simulink model "algeEquation"  (R2024b)
settings: Solver=VariableStepAuto  StartTime=0.0  StopTime=10.0  RelTol=1e-3
values from neighbouring files (symbols this model uses):
  m = input("enter the value for slop(m): ")    [algeEquMfile.m]
libraries: simulink x1
settings Model: Creator=admin  LastModifiedBy=admin

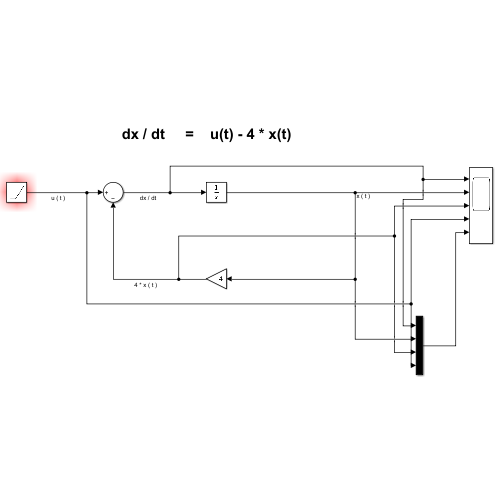
[thumbnail: Simulink's stored preview of the top-level diagram]
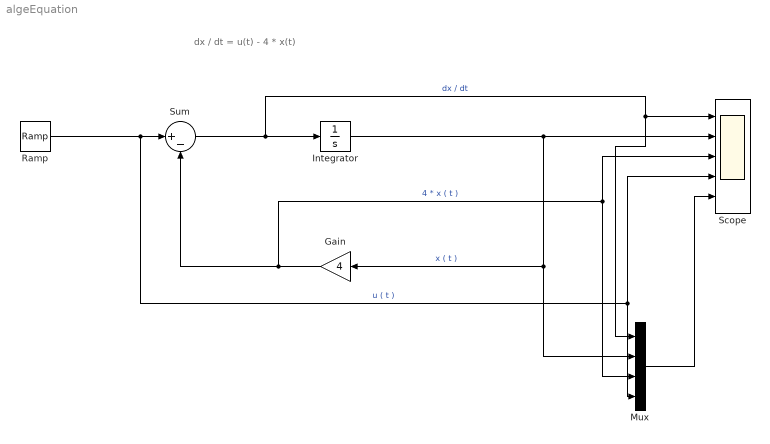
== system algeEquation ==
  note: dx / dt = u(t) - 4 * x(t)
  Gain : Gain  Gain=4
  Integrator : Integrator
  Mux : Mux
  Ramp : simulink/Sources/Ramp  slope=m  start=0  InitialOutput=0
  Scope : Scope  NumInputPorts=5
  Sum : Sum  Inputs=|+-
  wires:
  Sum/1 -> Mux/1, Scope/1, Integrator/1  "dx / dt"
  Ramp/1 -> Mux/4, Scope/4, Sum/1  "u ( t )"
  Integrator/1 -> Mux/2, Gain/1, Scope/2  "x ( t )"
  Gain/1 -> Mux/3, Scope/3, Sum/2  "4 * x ( t )"
  Mux/1 -> Scope/5
